simulink model "lab4_1"  (R2020b)
settings: Solver=VariableStepAuto  StartTime=0.0  StopTime=50  MaxStep=0.01  RelTol=1e-3
InitFcn:
  | a0 = 2;
  | a1 = -5;
  | b0 = 5;
  | A = [0 1; -a0 -a1];
  | b = [0; b0];
  | 
  | am0 = 64;
  | am1 = 16;
  | Am = [0 1; -am0 -am1];
  | bm = [0; am0];
  | 
  | theta1 = (a0 - am0)/b0;
  | theta2 = (a1 - am1)/b0;
  | kappa = b0/am0;
  | 
  | Q = eye(2);
  | P = lyap(Am', Q);
settings Model: Creator=Eeer12  LastModifiedBy=Eugene

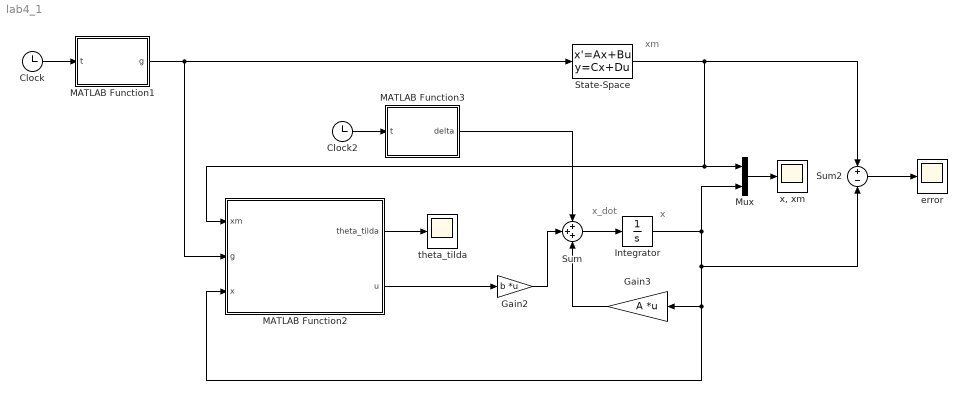
== system lab4_1 ==
  note: x_dot
  note: x
  note: xm
  Clock : Clock
  Clock2 : Clock
  Gain2 : Gain  Gain=b  Multiplication=Matrix(K*u)
  Gain3 : Gain  Gain=A  Multiplication=Matrix(K*u)
  Integrator : Integrator  InitialCondition=[0; 0]
  MATLAB Function1 : MATLAB Function  TreatAsAtomicUnit=on
  MATLAB Function2 : MATLAB Function  TreatAsAtomicUnit=on
  MATLAB Function3 : MATLAB Function  TreatAsAtomicUnit=on
  Mux : Mux  Inputs=2
  State-Space : StateSpace  A=Am  B=bm  C=eye(2)  D=[0; 0]  InitialCondition=[0; 0]
  Sum : Sum  Inputs=+++
  Sum2 : Sum  Inputs=+-
  error : Scope
  theta_tilda : Scope
  "x, xm" : Scope
  wires:
  Integrator/1 -> Mux/2, Gain3/1, MATLAB Function2/3(x), Sum2/2
  Sum/1 -> Integrator/1
  Clock/1 -> MATLAB Function1/1(t)
  MATLAB Function1/1(g) -> State-Space/1, MATLAB Function2/2(g)
  Gain3/1 -> Sum/3
  MATLAB Function2/2(u) -> Gain2/1
  Sum2/1 -> error/1
  MATLAB Function2/1(theta_tilda) -> theta_tilda/1
  State-Space/1 -> Sum2/1, Mux/1, MATLAB Function2/1(xm)
  Gain2/1 -> Sum/2
  Clock2/1 -> MATLAB Function3/1(t)
  MATLAB Function3/1(delta) -> Sum/1
  Mux/1 -> "x, xm"/1

== matlab function lab4_1/MATLAB Function1 ==
  data: t input; g output
function g = fcn(t)

g = 10*cos(0.5*t) + 2*sin(t) + 12;

== matlab function lab4_1/MATLAB Function2 ==
  data: xm input; theta_tilda output; g input; x input; u output; theta1 parameter; theta2 parameter; P parameter; kappa parameter; b parameter
function [theta_tilda, u] = fcn(xm, g, x, theta1, theta2, P, kappa, b)

theta = [theta1; theta2];
gamma = 5;
e = xm - x;
theta_hat = gamma*x*b'*P*e;
u = theta_hat'*x + g/kappa;
theta_tilda = theta - theta_hat;

== matlab function lab4_1/MATLAB Function3 ==
  data: t input; delta output
function delta = fcn(t)

delta = [0.6*sin(10*t) + 0.1*sin(50*t); 0.5*cos(12*t) + 0.2*sin(30*t)];
